simulink model "si1_matlabFcn"  (R2021b)
settings: Solver=VariableStepAuto  StartTime=0.0  StopTime=10.0  RelTol=1e-3
undefined symbols (not defined in the file or in its folder): A, f, phi
settings Model: Creator=sar  LastModifiedBy=sar
settings SolverCC: AlgebraicLoopSolver=TrustRegion
settings DataIOCC: Refine=10
settings DebuggingCC: SFMachineParentedDataDiag=warning

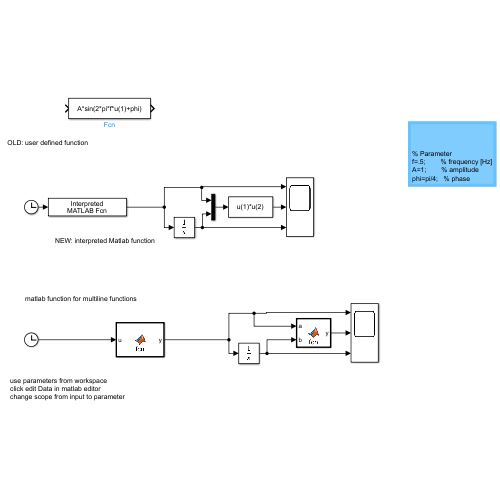
[thumbnail: Simulink's stored preview of the top-level diagram]
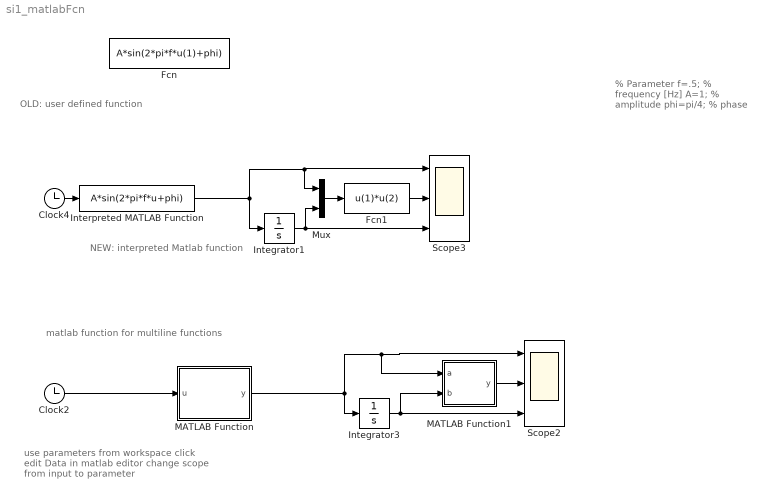
== system si1_matlabFcn ==
  note: NEW: interpreted Matlab function
  note: matlab function for multiline functions
  note: use parameters from workspace
      | click edit Data in matlab editor
      | change scope from input to parameter
  note: OLD: user defined function
  note: % Parameter
      | f=.5; % frequency [Hz]
      | A=1; % amplitude
      | phi=pi/4; % phase
  Clock2 : Clock
  Clock4 : Clock
  Fcn : Fcn  Expr=A*sin(2*pi*f*u(1)+phi)
  Fcn1 : Fcn  Expr=u(1)*u(2)
  Integrator1 : Integrator
  Integrator3 : Integrator
  Interpreted MATLAB Function : MATLABFcn  MATLABFcn=A*sin(2*pi*f*u+phi)
  MATLAB Function : MATLAB Function  TreatAsAtomicUnit=on
  MATLAB Function1 : MATLAB Function  TreatAsAtomicUnit=on
  Mux : Mux  Inputs=2
  Scope2 : Scope  NumInputPorts=3
  Scope3 : Scope  NumInputPorts=3
  wires:
  Integrator1/1 -> Mux/2, Scope3/3
  Fcn1/1 -> Scope3/2
  Mux/1 -> Fcn1/1
  Clock4/1 -> Interpreted MATLAB Function/1
  Interpreted MATLAB Function/1 -> Mux/1, Scope3/1, Integrator1/1
  MATLAB Function1/1(y) -> Scope2/2
  Integrator3/1 -> MATLAB Function1/2(b), Scope2/3
  MATLAB Function/1(y) -> Scope2/1, MATLAB Function1/1(a), Integrator3/1
  Clock2/1 -> MATLAB Function/1(u)

== matlab function si1_matlabFcn/MATLAB Function ==
  data: u input; y output; A parameter; phi parameter
function y = fcn(u, A, phi)
f=.5;        % Frequenz [Hz]

y = A*sin(2*pi*f*u+phi);

== matlab function si1_matlabFcn/MATLAB Function1 ==
  data: a input; y output; b input
function y = fcn(a,b)


y = a*b;
